simulink model "robotarm_generalization_error"  (R2018b)
settings: Solver=FixedStepAuto  StartTime=0.0  StopTime=10  FixedStep=options.dt  RelTol=1e-3  AbsTol=1e-6
PreLoadFcn:
  | const_ref=-0.1;
  | options.dt=0.02;
libraries: neural x528, simulink x1
(part 12 of 20)

== system robotarm_generalization_error/pre_0.00003/Layer 3/Delays 1 ==
  "p{3}" : Inport  PortDimensions=30
      mask Display: e = 0.06;c1 = [120 230 180]/255;c2 = ([120 230 180]+0)/(256+128);c3 = ([120 230 180]+128)/(256+128);patch([0 1 1 0],[0 0 1 1],c1);patch([0 1 1 1-e 1-e 0+e],[0 0 1 1-e 0+e 0+e],c2);patch([0 0 1 1-e 0+e 0+e],[0 1 1 1-e 1-e 0+e],c3);plot([0 1 1 0 0],[0 0 1 1 0]);
  mux : Mux  Inputs=1
      mask Display: e = 0.06;c1 = [120 150 230]/255;c2 = ([120 150 230]+0)/383;c3 = ([120 150 230]+128)/383;patch([0 1 1 0],[0 0 1 1],c1);patch([0 1 1 1-e 1-e 0+e],[0 0 1 1-e 0+e 0+e],c2);patch([0 0 1 1-e 0+e 0+e],[0 1 1 1-e 1-e 0+e],c3);plot([0 1 1 0 0],[0 0 1 1 0]);disp('Mux')
  "pd{3,2}" : Outport
      mask Display: e = 0.06;c1 = [120 230 180]/255;c2 = ([120 230 180]+0)/(256+128);c3 = ([120 230 180]+128)/(256+128);patch([0 1 1 0],[0 0 1 1],c1);patch([0 1 1 1-e 1-e 0+e],[0 0 1 1-e 0+e 0+e],c2);patch([0 0 1 1-e 0+e 0+e],[0 1 1 1-e 1-e 0+e],c3);plot([0 1 1 0 0],[0 0 1 1 0]);
  wires:
  "p{3}"/1 -> mux/1
  mux/1 -> "pd{3,2}"/1

== system robotarm_generalization_error/pre_0.00003/Layer 3/LW{3,2} ==
  "ad{3,2}" : Inport  PortDimensions=30
      mask Display: e = 0.06;c1 = [120 230 180]/255;c2 = ([120 230 180]+0)/(256+128);c3 = ([120 230 180]+128)/(256+128);patch([0 1 1 0],[0 0 1 1],c1);patch([0 1 1 1-e 1-e 0+e],[0 0 1 1-e 0+e 0+e],c2);patch([0 0 1 1-e 0+e 0+e],[0 1 1 1-e 1-e 0+e],c3);plot([0 1 1 0 0],[0 0 1 1 0]);
  "IW{3,2}(1,:)'" : Constant  Value=[0.364651980007638709668782439621281810104846954345703125;0.09359729132947780527729264576919376850128173828125;0.39849585177361046550714718250674195587635040283203125;0.483299133160862981473115951303043402731418609619140625;0.76043527816801514962463670599390752613544464111328125;0.123709877455670358425976473881746642291545867919921875;0.305627616621842845834322588416398502886295318603515625;-0.0626512881320664127837716250724042765796184539794921875;0.481490039958100746186886453870101831853389739990234375;-0.466397969762965491913320192907121963798999786376953125;0.108573478888505048356449833590886555612087249755859375;0.64413157489343320083463595437933690845966339111328125;0.26516202150267620396562051610089838504791259765625;0.291385173164447175420121993738575838506221771240234375;0.154484703639592935164870368680567480623722076416015625;-0.11628020441549259678115646465812460519373416900634765625;0.130705045350562321093690343332127667963504791259765625;0.192091777253844908646129852058948017656803131103515625;0.1613262484268893348637874396445113234221935272216796875;-0.064889250348107718746604177795234136283397674560546875;-0.28878754918844051768900271781603805720806121826171875;-0.1256166981918040992383112097741104662418365478515625;0.441166621361597066641735409575630910694599151611328125;-0.434871229251801050263992465261253528296947479248046875;0.25102983328520400707617454827413894236087799072265625;-0.1549482851295911067790456172588164918124675750732421875;0.339046773906632292749918633489869534969329833984375;-0.354977509945755997922134383770753629505634307861328125;-0.3983372866802117329143584356643259525299072265625;0.348439733827424602541356080109835602343082427978515625]
      mask Display: e = 0.06;c1 = [120 150 230]/255;c2 = ([120 150 230]+0)/383;c3 = ([120 150 230]+128)/383;patch([0 1 1 0],[0 0 1 1],c1);patch([0 1 1 1-e 1-e 0+e],[0 0 1 1-e 0+e 0+e],c2);patch([0 0 1 1-e 0+e 0+e],[0 1 1 1-e 1-e 0+e],c3);plot([0 1 1 0 0],[0 0 1 1 0]);disp('weights');
  Mux : Mux  Inputs=1
      mask Display: e = 0.06;c1 = [120 150 230]/255;c2 = ([120 150 230]+0)/383;c3 = ([120 150 230]+128)/383;patch([0 1 1 0],[0 0 1 1],c1);patch([0 1 1 1-e 1-e 0+e],[0 0 1 1-e 0+e 0+e],c2);patch([0 0 1 1-e 0+e 0+e],[0 1 1 1-e 1-e 0+e],c3);plot([0 1 1 0 0],[0 0 1 1 0]);disp('Mux');
  dotprod1 : neural/Weight Functions/dotprod
  "lz{3,2}" : Outport
      mask Display: e = 0.06;c1 = [120 230 180]/255;c2 = ([120 230 180]+0)/(256+128);c3 = ([120 230 180]+128)/(256+128);patch([0 1 1 0],[0 0 1 1],c1);patch([0 1 1 1-e 1-e 0+e],[0 0 1 1-e 0+e 0+e],c2);patch([0 0 1 1-e 0+e 0+e],[0 1 1 1-e 1-e 0+e],c3);plot([0 1 1 0 0],[0 0 1 1 0]);
  wires:
  "IW{3,2}(1,:)'"/1 -> dotprod1/1
  "ad{3,2}"/1 -> dotprod1/2
  dotprod1/1 -> Mux/1
  Mux/1 -> "lz{3,2}"/1

== system robotarm_generalization_error/pre_0.00004/Layer 1/Delays 1 ==
  "p{1}" : Inport  PortDimensions=10
      mask Display: e = 0.06;c1 = [120 230 180]/255;c2 = ([120 230 180]+0)/(256+128);c3 = ([120 230 180]+128)/(256+128);patch([0 1 1 0],[0 0 1 1],c1);patch([0 1 1 1-e 1-e 0+e],[0 0 1 1-e 0+e 0+e],c2);patch([0 0 1 1-e 0+e 0+e],[0 1 1 1-e 1-e 0+e],c3);plot([0 1 1 0 0],[0 0 1 1 0]);
  mux : Mux  Inputs=1
      mask Display: e = 0.06;c1 = [120 150 230]/255;c2 = ([120 150 230]+0)/383;c3 = ([120 150 230]+128)/383;patch([0 1 1 0],[0 0 1 1],c1);patch([0 1 1 1-e 1-e 0+e],[0 0 1 1-e 0+e 0+e],c2);patch([0 0 1 1-e 0+e 0+e],[0 1 1 1-e 1-e 0+e],c3);plot([0 1 1 0 0],[0 0 1 1 0]);disp('Mux')
  "pd{1,1}" : Outport
      mask Display: e = 0.06;c1 = [120 230 180]/255;c2 = ([120 230 180]+0)/(256+128);c3 = ([120 230 180]+128)/(256+128);patch([0 1 1 0],[0 0 1 1],c1);patch([0 1 1 1-e 1-e 0+e],[0 0 1 1-e 0+e 0+e],c2);patch([0 0 1 1-e 0+e 0+e],[0 1 1 1-e 1-e 0+e],c3);plot([0 1 1 0 0],[0 0 1 1 0]);
  wires:
  "p{1}"/1 -> mux/1
  mux/1 -> "pd{1,1}"/1

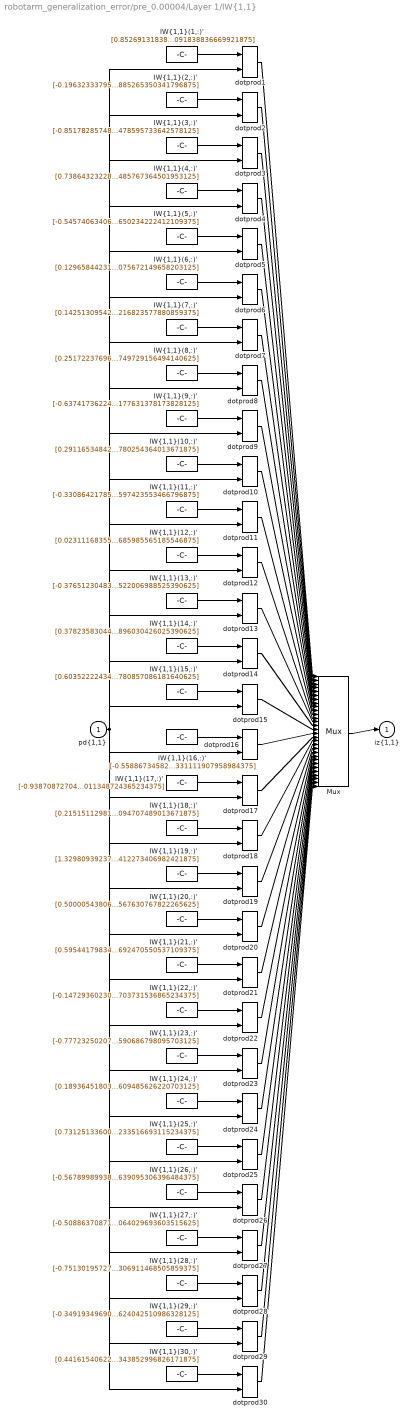
== system robotarm_generalization_error/pre_0.00004/Layer 1/IW{1,1} ==
  "pd{1,1}" : Inport  PortDimensions=10
      mask Display: e = 0.06;c1 = [120 230 180]/255;c2 = ([120 230 180]+0)/(256+128);c3 = ([120 230 180]+128)/(256+128);patch([0 1 1 0],[0 0 1 1],c1);patch([0 1 1 1-e 1-e 0+e],[0 0 1 1-e 0+e 0+e],c2);patch([0 0 1 1-e 0+e 0+e],[0 1 1 1-e 1-e 0+e],c3);plot([0 1 1 0 0],[0 0 1 1 0]);
  "IW{1,1}(1,:)'" : Constant  Value=[0.85269131838291956082542810690938495099544525146484375;0.841981756605793663084114086814224720001220703125;0.331962437287081801873256381441024132072925567626953125;0.27525840899203724010391169940703548491001129150390625;0.73414190805789047988838547098566778004169464111328125;-0.1787371875469097037836263552890159189701080322265625;0.653768958712303227542861350229941308498382568359375;0.331173327192727684487039141458808444440364837646484375;0.88652828404312611354498585569672286510467529296875;0.166520380073901186346319036601926200091838836669921875]
      mask Display: e = 0.06;c1 = [120 150 230]/255;c2 = ([120 150 230]+0)/383;c3 = ([120 150 230]+128)/383;patch([0 1 1 0],[0 0 1 1],c1);patch([0 1 1 1-e 1-e 0+e],[0 0 1 1-e 0+e 0+e],c2);patch([0 0 1 1-e 0+e 0+e],[0 1 1 1-e 1-e 0+e],c3);plot([0 1 1 0 0],[0 0 1 1 0]);disp('Weights');
  "IW{1,1}(10,:)'" : Constant  Value=[0.291165348423945591349593087215907871723175048828125;-0.722630551736977988497301339521072804927825927734375;-0.383989918106309724432634311597212217748165130615234375;0.46974786901538212458007137684035114943981170654296875;0.94282878770446731930832129364716820418834686279296875;-1.7095692356157392577387099663610570132732391357421875;1.1191750512147529139639345885370858013629913330078125;0.327709122006033137797231802323949523270130157470703125;-0.07377869006224868630994251361698843538761138916015625;-0.439984949358797450269520368237863294780254364013671875]
      mask Display: e = 0.06;c1 = [120 150 230]/255;c2 = ([120 150 230]+0)/383;c3 = ([120 150 230]+128)/383;patch([0 1 1 0],[0 0 1 1],c1);patch([0 1 1 1-e 1-e 0+e],[0 0 1 1-e 0+e 0+e],c2);patch([0 0 1 1-e 0+e 0+e],[0 1 1 1-e 1-e 0+e],c3);plot([0 1 1 0 0],[0 0 1 1 0]);disp('Weights');
  "IW{1,1}(11,:)'" : Constant  Value=[-0.33086421785925856919874377126689068973064422607421875;0.936860885950881794315137085504829883575439453125;-0.95620177422050656179663974398863501846790313720703125;-0.322294935271898286277547640565899200737476348876953125;0.68993221439925600524389892598264850676059722900390625;-0.5926530783861763129749533618451096117496490478515625;0.237770762895108289658452349613071419298648834228515625;0.4455800520287784838302513890084810554981231689453125;-0.290696552862368007286164584002108313143253326416015625;-0.7323399346148409261303413586574606597423553466796875]
      mask Display: e = 0.06;c1 = [120 150 230]/255;c2 = ([120 150 230]+0)/383;c3 = ([120 150 230]+128)/383;patch([0 1 1 0],[0 0 1 1],c1);patch([0 1 1 1-e 1-e 0+e],[0 0 1 1-e 0+e 0+e],c2);patch([0 0 1 1-e 0+e 0+e],[0 1 1 1-e 1-e 0+e],c3);plot([0 1 1 0 0],[0 0 1 1 0]);disp('Weights');
  "IW{1,1}(12,:)'" : Constant  Value=[0.0231116835533762450538564081625736434943974018096923828125;0.75724627159166779666321644981508143246173858642578125;0.169039308468649840389019800568348728120326995849609375;0.176165759180306025211137921360204927623271942138671875;-2.421132161938288618330261670053005218505859375;1.6872752903373917643392587706330232322216033935546875;-0.159214365090671272628952692684833891689777374267578125;-0.1720265892136304264337098857140517793595790863037109375;-0.4360980492722419388229582182248122990131378173828125;0.25290831940400249067124605062417685985565185546875]
      mask Display: e = 0.06;c1 = [120 150 230]/255;c2 = ([120 150 230]+0)/383;c3 = ([120 150 230]+128)/383;patch([0 1 1 0],[0 0 1 1],c1);patch([0 1 1 1-e 1-e 0+e],[0 0 1 1-e 0+e 0+e],c2);patch([0 0 1 1-e 0+e 0+e],[0 1 1 1-e 1-e 0+e],c3);plot([0 1 1 0 0],[0 0 1 1 0]);disp('Weights');
  "IW{1,1}(13,:)'" : Constant  Value=[-0.376512304837161415616009207951719872653484344482421875;-1.2243256163438112071872865271870978176593780517578125;0.9832341208016845968131747213192284107208251953125;0.54046742893889898606829547134111635386943817138671875;-0.10030983433967317897117510483440128155052661895751953125;0.2040299409647271244860888828043243847787380218505859375;-0.514657840634743291019503885763697326183319091796875;-0.308496361506203076174870147951878607273101806640625;-0.658101985059666549915391442482359707355499267578125;0.390982737869508378825145200607948936522006988525390625]
      mask Display: e = 0.06;c1 = [120 150 230]/255;c2 = ([120 150 230]+0)/383;c3 = ([120 150 230]+128)/383;patch([0 1 1 0],[0 0 1 1],c1);patch([0 1 1 1-e 1-e 0+e],[0 0 1 1-e 0+e 0+e],c2);patch([0 0 1 1-e 0+e 0+e],[0 1 1 1-e 1-e 0+e],c3);plot([0 1 1 0 0],[0 0 1 1 0]);disp('Weights');
  "IW{1,1}(14,:)'" : Constant  Value=[0.378235830447926579811479541604057885706424713134765625;-0.188578127409249785007006039450061507523059844970703125;0.89766484900875098684736030918429605662822723388671875;-0.012990602010364289686794592171281692571938037872314453125;-1.528037758353024688773302841582335531711578369140625;-0.684010049710931156141668907366693019866943359375;0.57024411656892637356719433228136040270328521728515625;-0.43202952191774401935475680147646926343441009521484375;-0.6718007028416217440991431431029923260211944580078125;0.342484082791047195204470199314528144896030426025390625]
      mask Display: e = 0.06;c1 = [120 150 230]/255;c2 = ([120 150 230]+0)/383;c3 = ([120 150 230]+128)/383;patch([0 1 1 0],[0 0 1 1],c1);patch([0 1 1 1-e 1-e 0+e],[0 0 1 1-e 0+e 0+e],c2);patch([0 0 1 1-e 0+e 0+e],[0 1 1 1-e 1-e 0+e],c3);plot([0 1 1 0 0],[0 0 1 1 0]);disp('Weights');
  "IW{1,1}(15,:)'" : Constant  Value=[0.6035222243453437496185642885393463075160980224609375;0.031586677444605283648915161620607250370085239410400390625;0.28267467967502302172988493111915886402130126953125;0.1996393263369853621203020566099439747631549835205078125;1.3525996950626069104117732422309927642345428466796875;-1.696130378060912047288866233429871499538421630859375;0.2202755721801854249530805418544332496821880340576171875;-0.2386512481300608612411195963431964628398418426513671875;0.1698997692033973605507668480640859343111515045166015625;0.57761542879031824160307451165863312780857086181640625]
      mask Display: e = 0.06;c1 = [120 150 230]/255;c2 = ([120 150 230]+0)/383;c3 = ([120 150 230]+128)/383;patch([0 1 1 0],[0 0 1 1],c1);patch([0 1 1 1-e 1-e 0+e],[0 0 1 1-e 0+e 0+e],c2);patch([0 0 1 1-e 0+e 0+e],[0 1 1 1-e 1-e 0+e],c3);plot([0 1 1 0 0],[0 0 1 1 0]);disp('Weights');
  "IW{1,1}(16,:)'" : Constant  Value=[-0.5588673458279860284392270841635763645172119140625;0.298136361747344091899236673270934261381626129150390625;0.78495094628481798526564716667053289711475372314453125;0.485471500839177949604419382012565620243549346923828125;1.4207066862265362860995310256839729845523834228515625;0.07462999056671358599768240082994452677667140960693359375;0.39795181740876639508996959193609654903411865234375;-0.83430821719863790253413071695831604301929473876953125;-1.0243906954380557206008006687625311315059661865234375;0.443779142565702444667152803958742879331111907958984375]
      mask Display: e = 0.06;c1 = [120 150 230]/255;c2 = ([120 150 230]+0)/383;c3 = ([120 150 230]+128)/383;patch([0 1 1 0],[0 0 1 1],c1);patch([0 1 1 1-e 1-e 0+e],[0 0 1 1-e 0+e 0+e],c2);patch([0 0 1 1-e 0+e 0+e],[0 1 1 1-e 1-e 0+e],c3);plot([0 1 1 0 0],[0 0 1 1 0]);disp('Weights');
  "IW{1,1}(17,:)'" : Constant  Value=[-0.9387087270454552712095619426690973341464996337890625;-0.89521919886691170287207341971225105226039886474609375;-0.0955800124964277519890032408511615358293056488037109375;-0.470995956174425856044507554543088190257549285888671875;-0.740778073100817113783023160067386925220489501953125;-1.394169789397575076606017319136299192905426025390625;0.76984119013535645681400865214527584612369537353515625;-0.53846772655583519107125312075368128716945648193359375;1.031008587153705580163887134403921663761138916015625;0.131779807710906859963273518587811850011348724365234375]
      mask Display: e = 0.06;c1 = [120 150 230]/255;c2 = ([120 150 230]+0)/383;c3 = ([120 150 230]+128)/383;patch([0 1 1 0],[0 0 1 1],c1);patch([0 1 1 1-e 1-e 0+e],[0 0 1 1-e 0+e 0+e],c2);patch([0 0 1 1-e 0+e 0+e],[0 1 1 1-e 1-e 0+e],c3);plot([0 1 1 0 0],[0 0 1 1 0]);disp('Weights');
  "IW{1,1}(18,:)'" : Constant  Value=[0.215151129816157415941546560134156607091426849365234375;0.038882851458689131340928923918909276835620403289794921875;1.5800118154952988991368556526140309870243072509765625;-0.469405682176665506322166265817941166460514068603515625;0.9294512492106061785079873516224324703216552734375;-0.719382127872345566999001675867475569248199462890625;0.5627218358246575125036770259612239897251129150390625;0.804486287135425914840425321017391979694366455078125;1.1217948675047584305985992614296264946460723876953125;0.2403996058936139490480599079091916792094707489013671875]
      mask Display: e = 0.06;c1 = [120 150 230]/255;c2 = ([120 150 230]+0)/383;c3 = ([120 150 230]+128)/383;patch([0 1 1 0],[0 0 1 1],c1);patch([0 1 1 1-e 1-e 0+e],[0 0 1 1-e 0+e 0+e],c2);patch([0 0 1 1-e 0+e 0+e],[0 1 1 1-e 1-e 0+e],c3);plot([0 1 1 0 0],[0 0 1 1 0]);disp('Weights');
  "IW{1,1}(19,:)'" : Constant  Value=[1.3298093923795162307754935682169161736965179443359375;-0.333531558196221766809941300380160100758075714111328125;0.05092309669358834056662743705601315014064311981201171875;0.08687966425010419657670723836417892016470432281494140625;0.188629616681764422647660239817923866212368011474609375;0.62559182702411508802953221675124950706958770751953125;0.94268254803254480922447555713006295263767242431640625;-0.378498913515795953887987934649572707712650299072265625;0.65036328382864472263946709063020534813404083251953125;0.68436573878344908461457407611305825412273406982421875]
      mask Display: e = 0.06;c1 = [120 150 230]/255;c2 = ([120 150 230]+0)/383;c3 = ([120 150 230]+128)/383;patch([0 1 1 0],[0 0 1 1],c1);patch([0 1 1 1-e 1-e 0+e],[0 0 1 1-e 0+e 0+e],c2);patch([0 0 1 1-e 0+e 0+e],[0 1 1 1-e 1-e 0+e],c3);plot([0 1 1 0 0],[0 0 1 1 0]);disp('Weights');
  "IW{1,1}(2,:)'" : Constant  Value=[-0.1963233379558946001264274627828854136168956756591796875;1.101305050049736333761529749608598649501800537109375;0.311527646283544623617700608519953675568103790283203125;-0.3416615891814156480421615924569778144359588623046875;0.638619513911475422673902357928454875946044921875;0.138176661634680508772277107709669508039951324462890625;-0.3473382142907117664520910693681798875331878662109375;-0.409370711295091449510863412797334603965282440185546875;1.162931446196200813147925146040506660938262939453125;0.63642421861614184575017816314357332885265350341796875]
      mask Display: e = 0.06;c1 = [120 150 230]/255;c2 = ([120 150 230]+0)/383;c3 = ([120 150 230]+128)/383;patch([0 1 1 0],[0 0 1 1],c1);patch([0 1 1 1-e 1-e 0+e],[0 0 1 1-e 0+e 0+e],c2);patch([0 0 1 1-e 0+e 0+e],[0 1 1 1-e 1-e 0+e],c3);plot([0 1 1 0 0],[0 0 1 1 0]);disp('Weights');
  "IW{1,1}(20,:)'" : Constant  Value=[0.500005438060606710592992385500110685825347900390625;0.32554598125672618014192494229064323008060455322265625;0.05401003034234606869912198590100160799920558929443359375;-0.328993966207549781710639535958762280642986297607421875;0.90299818716244717453633938930579461157321929931640625;-1.81145213752210576529932950506918132305145263671875;1.1771176901383146873314444746938534080982208251953125;0.14858704542182110674986006415565498173236846923828125;0.2082982131750723275853687255221302621066570281982421875;0.54042026994425163000101974830613471567630767822265625]
      mask Display: e = 0.06;c1 = [120 150 230]/255;c2 = ([120 150 230]+0)/383;c3 = ([120 150 230]+128)/383;patch([0 1 1 0],[0 0 1 1],c1);patch([0 1 1 1-e 1-e 0+e],[0 0 1 1-e 0+e 0+e],c2);patch([0 0 1 1-e 0+e 0+e],[0 1 1 1-e 1-e 0+e],c3);plot([0 1 1 0 0],[0 0 1 1 0]);disp('Weights');
  "IW{1,1}(21,:)'" : Constant  Value=[0.59544179834568156106655578696518205106258392333984375;-0.58314726685634321601270357859903015196323394775390625;-0.1664517788060776715131083847154513932764530181884765625;-0.43602397923763069886859966572956182062625885009765625;-0.3105195838993994872367920834221877157688140869140625;0.5996396338687419724777782903402112424373626708984375;-0.09051775044418723659145342708143289200961589813232421875;0.257824502565505209172869172107311896979808807373046875;0.39321157589385891117927940285881049931049346923828125;1.0959331280914508255364125943742692470550537109375]
      mask Display: e = 0.06;c1 = [120 150 230]/255;c2 = ([120 150 230]+0)/383;c3 = ([120 150 230]+128)/383;patch([0 1 1 0],[0 0 1 1],c1);patch([0 1 1 1-e 1-e 0+e],[0 0 1 1-e 0+e 0+e],c2);patch([0 0 1 1-e 0+e 0+e],[0 1 1 1-e 1-e 0+e],c3);plot([0 1 1 0 0],[0 0 1 1 0]);disp('Weights');
  "IW{1,1}(22,:)'" : Constant  Value=[-0.1472936023089768953209244273239164613187313079833984375;-0.441888252579368978611995544270030222833156585693359375;-0.30245270098367205147127378950244747102260589599609375;0.6369811429104677014123581102467142045497894287109375;0.150084332027071665205397721365443430840969085693359375;0.28010115984977945746692284956225194036960601806640625;0.70947230228804603058279099059291183948516845703125;-0.51608692547304169107036386776599101722240447998046875;0.413275589919472607913775163979153148829936981201171875;-0.66863305601651157328291219528182409703731536865234375]
      mask Display: e = 0.06;c1 = [120 150 230]/255;c2 = ([120 150 230]+0)/383;c3 = ([120 150 230]+128)/383;patch([0 1 1 0],[0 0 1 1],c1);patch([0 1 1 1-e 1-e 0+e],[0 0 1 1-e 0+e 0+e],c2);patch([0 0 1 1-e 0+e 0+e],[0 1 1 1-e 1-e 0+e],c3);plot([0 1 1 0 0],[0 0 1 1 0]);disp('Weights');
  "IW{1,1}(23,:)'" : Constant  Value=[-0.7772325020715820098615722599788568913936614990234375;-0.89903016899141896534075613089953549206256866455078125;-0.84177580602092094697042057305225171148777008056640625;0.12045864842042598719107360238922410644590854644775390625;0.73296342722170793049230042015551589429378509521484375;0.2035185655751734490337412353255786001682281494140625;-0.2709032805624129736088434583507478237152099609375;-0.1758574275875861847584502584140864200890064239501953125;0.31969040218915256712506334224599413573741912841796875;0.292643085817043069329912441389751620590686798095703125]
      mask Display: e = 0.06;c1 = [120 150 230]/255;c2 = ([120 150 230]+0)/383;c3 = ([120 150 230]+128)/383;patch([0 1 1 0],[0 0 1 1],c1);patch([0 1 1 1-e 1-e 0+e],[0 0 1 1-e 0+e 0+e],c2);patch([0 0 1 1-e 0+e 0+e],[0 1 1 1-e 1-e 0+e],c3);plot([0 1 1 0 0],[0 0 1 1 0]);disp('Weights');
  "IW{1,1}(24,:)'" : Constant  Value=[0.1893645180384876114398906565838842652738094329833984375;-0.0270356922898101238728063577809734852053225040435791015625;-0.476109136040419544944057861357578076422214508056640625;-0.76440811123115126601845759068964980542659759521484375;-1.02375530684315219076552239130251109600067138671875;-2.0395759832134157107930150232277810573577880859375;0.7972269173860169200196423844317905604839324951171875;0.55158844103822091131661409235675819218158721923828125;0.59622552774299031330684783824835903942584991455078125;-0.01726826989945007273519195223343558609485626220703125]
      mask Display: e = 0.06;c1 = [120 150 230]/255;c2 = ([120 150 230]+0)/383;c3 = ([120 150 230]+128)/383;patch([0 1 1 0],[0 0 1 1],c1);patch([0 1 1 1-e 1-e 0+e],[0 0 1 1-e 0+e 0+e],c2);patch([0 0 1 1-e 0+e 0+e],[0 1 1 1-e 1-e 0+e],c3);plot([0 1 1 0 0],[0 0 1 1 0]);disp('Weights');
  "IW{1,1}(25,:)'" : Constant  Value=[0.73125133600929681509938973249518312513828277587890625;0.78572784904124082228094039237475953996181488037109375;0.464452230597018067559389464804553426802158355712890625;0.153547854639443925872654972408781759440898895263671875;0.51253755473311335411068512257770635187625885009765625;-0.63498210200908744571535180512000806629657745361328125;0.712270339038785227359085183707065880298614501953125;0.911310721932717004989399356418289244174957275390625;0.89225798461510386072603751017595641314983367919921875;-0.041150528524451744638579242518972023390233516693115234375]
      mask Display: e = 0.06;c1 = [120 150 230]/255;c2 = ([120 150 230]+0)/383;c3 = ([120 150 230]+128)/383;patch([0 1 1 0],[0 0 1 1],c1);patch([0 1 1 1-e 1-e 0+e],[0 0 1 1-e 0+e 0+e],c2);patch([0 0 1 1-e 0+e 0+e],[0 1 1 1-e 1-e 0+e],c3);plot([0 1 1 0 0],[0 0 1 1 0]);disp('Weights');
  "IW{1,1}(26,:)'" : Constant  Value=[-0.5678998993863491051570235867984592914581298828125;0.205165510402046280535870437233825214207172393798828125;-0.5239280884218475708991036299266852438449859619140625;0.71150802805785862137355479717371053993701934814453125;-0.021851450730236206265733045484012109227478504180908203125;0.08544806437122855202748183955918648280203342437744140625;0.53301147489959677105986202150234021246433258056640625;-0.97970664358083248135500298303668387234210968017578125;-0.1500014301673568140049752628328860737383365631103515625;-0.573092455164751157781211077235639095306396484375]
      mask Display: e = 0.06;c1 = [120 150 230]/255;c2 = ([120 150 230]+0)/383;c3 = ([120 150 230]+128)/383;patch([0 1 1 0],[0 0 1 1],c1);patch([0 1 1 1-e 1-e 0+e],[0 0 1 1-e 0+e 0+e],c2);patch([0 0 1 1-e 0+e 0+e],[0 1 1 1-e 1-e 0+e],c3);plot([0 1 1 0 0],[0 0 1 1 0]);disp('Weights');
  "IW{1,1}(27,:)'" : Constant  Value=[-0.508863708710330708839819635613821446895599365234375;0.08965567232304171019219296567825949750840663909912109375;-1.043231285850864775710533649544231593608856201171875;0.60319557825066205669628516261582262814044952392578125;0.5377687957246235495034625273547135293483734130859375;0.751181030100342095323640023707412183284759521484375;-0.212363215133831106928852250348427332937717437744140625;0.53687424858786114700848202119232155382633209228515625;0.272214509073961441476541267547872848808765411376953125;0.54452838894872412911496439846814610064029693603515625]
      mask Display: e = 0.06;c1 = [120 150 230]/255;c2 = ([120 150 230]+0)/383;c3 = ([120 150 230]+128)/383;patch([0 1 1 0],[0 0 1 1],c1);patch([0 1 1 1-e 1-e 0+e],[0 0 1 1-e 0+e 0+e],c2);patch([0 0 1 1-e 0+e 0+e],[0 1 1 1-e 1-e 0+e],c3);plot([0 1 1 0 0],[0 0 1 1 0]);disp('Weights');
  "IW{1,1}(28,:)'" : Constant  Value=[-0.75130195727908166691833002914790995419025421142578125;-0.32198020293129203661663950697402469813823699951171875;0.484451056801052437617016721560503356158733367919921875;0.71377872987490587064485225710086524486541748046875;0.70015196535886392581460313522256910800933837890625;-1.68264448928505938596345004043541848659515380859375;0.54789368678109884314153532614000141620635986328125;-0.15553292698856846509869455985608510673046112060546875;-0.2060856634002382337111924925920902751386165618896484375;-0.3000626849857821465406004790565930306911468505859375]
      mask Display: e = 0.06;c1 = [120 150 230]/255;c2 = ([120 150 230]+0)/383;c3 = ([120 150 230]+128)/383;patch([0 1 1 0],[0 0 1 1],c1);patch([0 1 1 1-e 1-e 0+e],[0 0 1 1-e 0+e 0+e],c2);patch([0 0 1 1-e 0+e 0+e],[0 1 1 1-e 1-e 0+e],c3);plot([0 1 1 0 0],[0 0 1 1 0]);disp('Weights');
  "IW{1,1}(29,:)'" : Constant  Value=[-0.349193496908300315961781734586111269891262054443359375;-0.395994643002482937799157980407471768558025360107421875;0.92539663473603261945044096137280575931072235107421875;0.12415477132418033245908617345776292495429515838623046875;0.300000619882113850334093285709968768060207366943359375;-1.15585511439208854511662138975225389003753662109375;-0.72933658912764964821207058776053600013256072998046875;-0.375071224928045177104962704106583259999752044677734375;-0.52071554481441195694202406230033375322818756103515625;-0.50971205825350296425568785707582719624042510986328125]
      mask Display: e = 0.06;c1 = [120 150 230]/255;c2 = ([120 150 230]+0)/383;c3 = ([120 150 230]+128)/383;patch([0 1 1 0],[0 0 1 1],c1);patch([0 1 1 1-e 1-e 0+e],[0 0 1 1-e 0+e 0+e],c2);patch([0 0 1 1-e 0+e 0+e],[0 1 1 1-e 1-e 0+e],c3);plot([0 1 1 0 0],[0 0 1 1 0]);disp('Weights');
  "IW{1,1}(3,:)'" : Constant  Value=[-0.85178285748256354903418241519830189645290374755859375;0.493601077255044040636988711412413977086544036865234375;0.30290787333167179529169743545935489237308502197265625;0.41544953946644380682329256160301156342029571533203125;1.1668049491410543705427471650182269513607025146484375;-0.787038886235399193225248382077552378177642822265625;-0.84781568094068815444330766695202328264713287353515625;-0.2947729693411724749552149660303257405757904052734375;0.438811116374599186062965827659354545176029205322265625;-0.248467595227088999809694769282941706478595733642578125]
      mask Display: e = 0.06;c1 = [120 150 230]/255;c2 = ([120 150 230]+0)/383;c3 = ([120 150 230]+128)/383;patch([0 1 1 0],[0 0 1 1],c1);patch([0 1 1 1-e 1-e 0+e],[0 0 1 1-e 0+e 0+e],c2);patch([0 0 1 1-e 0+e 0+e],[0 1 1 1-e 1-e 0+e],c3);plot([0 1 1 0 0],[0 0 1 1 0]);disp('Weights');
  "IW{1,1}(30,:)'" : Constant  Value=[0.441615406224214968045060913937049917876720428466796875;0.546337059731330842993202168145217001438140869140625;0.235248113230295319286966559957363642752170562744140625;-0.91108684930067507234952017824980430305004119873046875;1.3778962642149690243087434282642789185047149658203125;0.204095729606039666403916044146171770989894866943359375;0.08195113501367116970452997293250518850982189178466796875;-0.2543901485113078120292584571870975196361541748046875;0.55445717033132091433600407981430180370807647705078125;-0.00526920576212530460125105236102172057144343852996826171875]
      mask Display: e = 0.06;c1 = [120 150 230]/255;c2 = ([120 150 230]+0)/383;c3 = ([120 150 230]+128)/383;patch([0 1 1 0],[0 0 1 1],c1);patch([0 1 1 1-e 1-e 0+e],[0 0 1 1-e 0+e 0+e],c2);patch([0 0 1 1-e 0+e 0+e],[0 1 1 1-e 1-e 0+e],c3);plot([0 1 1 0 0],[0 0 1 1 0]);disp('Weights');
  "IW{1,1}(4,:)'" : Constant  Value=[0.73864323228570516466362505525466986000537872314453125;-0.523505647884718872120402011205442249774932861328125;0.3980804942710658433924209020915441215038299560546875;0.10753299151638516517603960664928308688104152679443359375;-1.1588546574510463216256539453752338886260986328125;0.8037395752259024472863302435143850743770599365234375;-0.5266235483237320380567325628362596035003662109375;0.07718309676004041219865570155889145098626613616943359375;-1.251443824189863107676501385867595672607421875;-0.157733727105185739247872334090061485767364501953125]
      mask Display: e = 0.06;c1 = [120 150 230]/255;c2 = ([120 150 230]+0)/383;c3 = ([120 150 230]+128)/383;patch([0 1 1 0],[0 0 1 1],c1);patch([0 1 1 1-e 1-e 0+e],[0 0 1 1-e 0+e 0+e],c2);patch([0 0 1 1-e 0+e 0+e],[0 1 1 1-e 1-e 0+e],c3);plot([0 1 1 0 0],[0 0 1 1 0]);disp('Weights');
  "IW{1,1}(5,:)'" : Constant  Value=[-0.54574063406632278283581172217964194715023040771484375;-0.9897782058903568103147563306265510618686676025390625;1.0857490928204998059669605936505831778049468994140625;-0.67493579564179728702555394193041138350963592529296875;-0.3846085993891030785363227550988085567951202392578125;0.1048413262275225132924560966785065829753875732421875;0.1100119495538010305768494845324312336742877960205078125;0.371119344710934218056763711501844227313995361328125;-0.5215011951386248068018858248251490294933319091796875;0.1526838773365060963893569123683846555650234222412109375]
      mask Display: e = 0.06;c1 = [120 150 230]/255;c2 = ([120 150 230]+0)/383;c3 = ([120 150 230]+128)/383;patch([0 1 1 0],[0 0 1 1],c1);patch([0 1 1 1-e 1-e 0+e],[0 0 1 1-e 0+e 0+e],c2);patch([0 0 1 1-e 0+e 0+e],[0 1 1 1-e 1-e 0+e],c3);plot([0 1 1 0 0],[0 0 1 1 0]);disp('Weights');
  "IW{1,1}(6,:)'" : Constant  Value=[0.1296584423152470633144872635966748930513858795166015625;0.03477824806126518508708755916813970543444156646728515625;-0.5581312920277670119872936993488110601902008056640625;-0.30117757438587577922817217768169939517974853515625;1.1171640309169159621660583070479333400726318359375;-1.8654965018841611623656717711128294467926025390625;0.82536280673833595233901405663345940411090850830078125;-0.469113198564734823481359171637450344860553741455078125;-0.2366428735693980323073759564067586325109004974365234375;0.14594072413917302810659748502075672149658203125]
      mask Display: e = 0.06;c1 = [120 150 230]/255;c2 = ([120 150 230]+0)/383;c3 = ([120 150 230]+128)/383;patch([0 1 1 0],[0 0 1 1],c1);patch([0 1 1 1-e 1-e 0+e],[0 0 1 1-e 0+e 0+e],c2);patch([0 0 1 1-e 0+e 0+e],[0 1 1 1-e 1-e 0+e],c3);plot([0 1 1 0 0],[0 0 1 1 0]);disp('Weights');
  "IW{1,1}(7,:)'" : Constant  Value=[0.1425130954232169677720065692483331076800823211669921875;1.2477174769943706333918953532702289521694183349609375;0.01841108366322040390539171994532807730138301849365234375;0.54900365251497784679912683714064769446849822998046875;0.0074865388773786671616772281367957475595176219940185546875;1.3852383664945537855572865737485699355602264404296875;0.219708070021052248588233624104759655892848968505859375;-0.26030212525183937799511113553307950496673583984375;-0.8235168113712261206416087588877417147159576416015625;-0.76161283143930302852453451123437844216823577880859375]
      mask Display: e = 0.06;c1 = [120 150 230]/255;c2 = ([120 150 230]+0)/383;c3 = ([120 150 230]+128)/383;patch([0 1 1 0],[0 0 1 1],c1);patch([0 1 1 1-e 1-e 0+e],[0 0 1 1-e 0+e 0+e],c2);patch([0 0 1 1-e 0+e 0+e],[0 1 1 1-e 1-e 0+e],c3);plot([0 1 1 0 0],[0 0 1 1 0]);disp('Weights');
  "IW{1,1}(8,:)'" : Constant  Value=[0.2517223769607410677195957759977318346500396728515625;-0.6150125546476326032774295526905916631221771240234375;0.7161158803491127766704948953702114522457122802734375;0.463508683499992690801860817373380996286869049072265625;0.61406160034275003578585483410279266536235809326171875;0.341264387354258236229043177445419132709503173828125;0.56339109255141917032005949295125901699066162109375;0.281055047926790868562108016703859902918338775634765625;-0.0277303153652980437227082433082614443264901638031005859375;0.6493460286010945825552198584773577749729156494140625]
      mask Display: e = 0.06;c1 = [120 150 230]/255;c2 = ([120 150 230]+0)/383;c3 = ([120 150 230]+128)/383;patch([0 1 1 0],[0 0 1 1],c1);patch([0 1 1 1-e 1-e 0+e],[0 0 1 1-e 0+e 0+e],c2);patch([0 0 1 1-e 0+e 0+e],[0 1 1 1-e 1-e 0+e],c3);plot([0 1 1 0 0],[0 0 1 1 0]);disp('Weights');
  "IW{1,1}(9,:)'" : Constant  Value=[-0.63741736224550049616510705163818784058094024658203125;0.74066610638293750579208563067368231713771820068359375;0.851058120001451090530508736264891922473907470703125;0.024530598551635245108126781587998266331851482391357421875;0.79001397863577327296269459111499600112438201904296875;1.3887123439372384137158178418758325278759002685546875;0.55185785354155247883767287930822931230068206787109375;-0.88747858851146921299601899590925313532352447509765625;-0.322743474582950884421705950444447807967662811279296875;-0.287853523327260163444663021437008865177631378173828125]
      mask Display: e = 0.06;c1 = [120 150 230]/255;c2 = ([120 150 230]+0)/383;c3 = ([120 150 230]+128)/383;patch([0 1 1 0],[0 0 1 1],c1);patch([0 1 1 1-e 1-e 0+e],[0 0 1 1-e 0+e 0+e],c2);patch([0 0 1 1-e 0+e 0+e],[0 1 1 1-e 1-e 0+e],c3);plot([0 1 1 0 0],[0 0 1 1 0]);disp('Weights');
  Mux : Mux  Inputs=30
      mask Display: e = 0.06;c1 = [120 150 230]/255;c2 = ([120 150 230]+0)/383;c3 = ([120 150 230]+128)/383;patch([0 1 1 0],[0 0 1 1],c1);patch([0 1 1 1-e 1-e 0+e],[0 0 1 1-e 0+e 0+e],c2);patch([0 0 1 1-e 0+e 0+e],[0 1 1 1-e 1-e 0+e],c3);plot([0 1 1 0 0],[0 0 1 1 0]);disp('Mux');
  dotprod{1..30} (30 alike) : neural/Weight Functions/dotprod
  "iz{1,1}" : Outport
      mask Display: e = 0.06;c1 = [120 230 180]/255;c2 = ([120 230 180]+0)/(256+128);c3 = ([120 230 180]+128)/(256+128);patch([0 1 1 0],[0 0 1 1],c1);patch([0 1 1 1-e 1-e 0+e],[0 0 1 1-e 0+e 0+e],c2);patch([0 0 1 1-e 0+e 0+e],[0 1 1 1-e 1-e 0+e],c3);plot([0 1 1 0 0],[0 0 1 1 0]);
  wires:
  "IW{1,1}(1,:)'"/1 -> dotprod1/1
  "pd{1,1}"/1 -> dotprod1/2, dotprod2/2, dotprod3/2, dotprod4/2, dotprod5/2, dotprod6/2, dotprod7/2, dotprod8/2, dotprod9/2, dotprod10/2, dotprod11/2, dotprod12/2, dotprod13/2, dotprod14/2, dotprod15/2, dotprod16/2, dotprod17/2, dotprod18/2, dotprod19/2, dotprod20/2, dotprod21/2, dotprod22/2, dotprod23/2, dotprod24/2, dotprod25/2, dotprod26/2, dotprod27/2, dotprod28/2, dotprod29/2, dotprod30/2
  dotprod1/1 -> Mux/1
  "IW{1,1}(2,:)'"/1 -> dotprod2/1
  dotprod2/1 -> Mux/2
  "IW{1,1}(3,:)'"/1 -> dotprod3/1
  dotprod3/1 -> Mux/3
  "IW{1,1}(4,:)'"/1 -> dotprod4/1
  dotprod4/1 -> Mux/4
  "IW{1,1}(5,:)'"/1 -> dotprod5/1
  dotprod5/1 -> Mux/5
  "IW{1,1}(6,:)'"/1 -> dotprod6/1
  dotprod6/1 -> Mux/6
  "IW{1,1}(7,:)'"/1 -> dotprod7/1
  dotprod7/1 -> Mux/7
  "IW{1,1}(8,:)'"/1 -> dotprod8/1
  dotprod8/1 -> Mux/8
  "IW{1,1}(9,:)'"/1 -> dotprod9/1
  dotprod9/1 -> Mux/9
  "IW{1,1}(10,:)'"/1 -> dotprod10/1
  dotprod10/1 -> Mux/10
  "IW{1,1}(11,:)'"/1 -> dotprod11/1
  dotprod11/1 -> Mux/11
  "IW{1,1}(12,:)'"/1 -> dotprod12/1
  dotprod12/1 -> Mux/12
  "IW{1,1}(13,:)'"/1 -> dotprod13/1
  dotprod13/1 -> Mux/13
  "IW{1,1}(14,:)'"/1 -> dotprod14/1
  dotprod14/1 -> Mux/14
  "IW{1,1}(15,:)'"/1 -> dotprod15/1
  dotprod15/1 -> Mux/15
  "IW{1,1}(16,:)'"/1 -> dotprod16/1
  dotprod16/1 -> Mux/16
  "IW{1,1}(17,:)'"/1 -> dotprod17/1
  dotprod17/1 -> Mux/17
  "IW{1,1}(18,:)'"/1 -> dotprod18/1
  dotprod18/1 -> Mux/18
  "IW{1,1}(19,:)'"/1 -> dotprod19/1
  dotprod19/1 -> Mux/19
  "IW{1,1}(20,:)'"/1 -> dotprod20/1
  dotprod20/1 -> Mux/20
  "IW{1,1}(21,:)'"/1 -> dotprod21/1
  dotprod21/1 -> Mux/21
  "IW{1,1}(22,:)'"/1 -> dotprod22/1
  dotprod22/1 -> Mux/22
  "IW{1,1}(23,:)'"/1 -> dotprod23/1
  dotprod23/1 -> Mux/23
  "IW{1,1}(24,:)'"/1 -> dotprod24/1
  dotprod24/1 -> Mux/24
  "IW{1,1}(25,:)'"/1 -> dotprod25/1
  dotprod25/1 -> Mux/25
  "IW{1,1}(26,:)'"/1 -> dotprod26/1
  dotprod26/1 -> Mux/26
  "IW{1,1}(27,:)'"/1 -> dotprod27/1
  dotprod27/1 -> Mux/27
  "IW{1,1}(28,:)'"/1 -> dotprod28/1
  dotprod28/1 -> Mux/28
  "IW{1,1}(29,:)'"/1 -> dotprod29/1
  dotprod29/1 -> Mux/29
  "IW{1,1}(30,:)'"/1 -> dotprod30/1
  dotprod30/1 -> Mux/30
  Mux/1 -> "iz{1,1}"/1

== system robotarm_generalization_error/pre_0.00004/Layer 2/Delays 1 ==
  "p{2}" : Inport  PortDimensions=30
      mask Display: e = 0.06;c1 = [120 230 180]/255;c2 = ([120 230 180]+0)/(256+128);c3 = ([120 230 180]+128)/(256+128);patch([0 1 1 0],[0 0 1 1],c1);patch([0 1 1 1-e 1-e 0+e],[0 0 1 1-e 0+e 0+e],c2);patch([0 0 1 1-e 0+e 0+e],[0 1 1 1-e 1-e 0+e],c3);plot([0 1 1 0 0],[0 0 1 1 0]);
  mux : Mux  Inputs=1
      mask Display: e = 0.06;c1 = [120 150 230]/255;c2 = ([120 150 230]+0)/383;c3 = ([120 150 230]+128)/383;patch([0 1 1 0],[0 0 1 1],c1);patch([0 1 1 1-e 1-e 0+e],[0 0 1 1-e 0+e 0+e],c2);patch([0 0 1 1-e 0+e 0+e],[0 1 1 1-e 1-e 0+e],c3);plot([0 1 1 0 0],[0 0 1 1 0]);disp('Mux')
  "pd{2,1}" : Outport
      mask Display: e = 0.06;c1 = [120 230 180]/255;c2 = ([120 230 180]+0)/(256+128);c3 = ([120 230 180]+128)/(256+128);patch([0 1 1 0],[0 0 1 1],c1);patch([0 1 1 1-e 1-e 0+e],[0 0 1 1-e 0+e 0+e],c2);patch([0 0 1 1-e 0+e 0+e],[0 1 1 1-e 1-e 0+e],c3);plot([0 1 1 0 0],[0 0 1 1 0]);
  wires:
  "p{2}"/1 -> mux/1
  mux/1 -> "pd{2,1}"/1
